simulink model "BFN_02_Thrusters"  (R2019b)
settings: Solver=VariableStepAuto  StartTime=0.0  StopTime=20  MaxStep=0.1  RelTol=1e-3
values from neighbouring files (symbols this model uses):
  MIB = 1e-3    (= 0.001)    [BFN_00_main.m]
  PWM_period = 0.1    [BFN_00_main.m]
  Thr_dir = [0 0 0 0 0 0 0 0 0 0 0 0;     0 0 1 -1 1 -1 0 0 1 -1 1 -1;     1 -1 0 0 0 0 1 -1 0 0 0 0]    [BFN_00_main.m]
  Thr_dist = [17 17 17 17 0 0 -17 -17 -17 -17 0 0;     0 0 0 0 0 0 0 0 0 0 0 0;     0 0 0 0 10 10 0 0 0 0 -10 -10]*1e-2    [BFN_00_main.m]
  Tmax = 500e-6    (= 0.0005)    [BFN_00_main.m]
  Tmin = 10e-6    (= 1e-05)    [BFN_00_main.m]
libraries: simulink x2
settings Model: Creator=Nicola  LastModifiedBy=Nicola

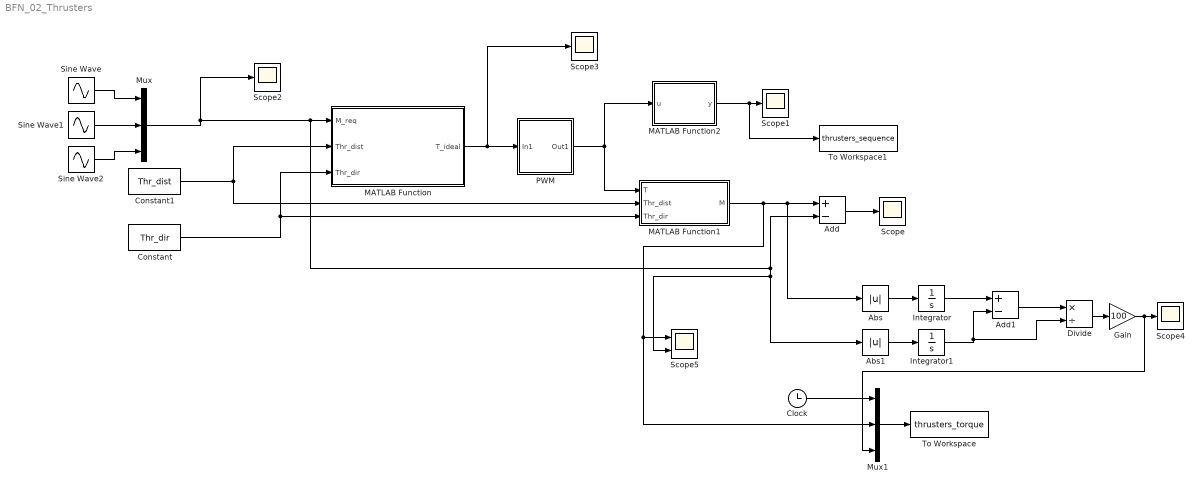
== system BFN_02_Thrusters ==
  Abs : Abs  ZeroCross=off
  Abs1 : Abs  ZeroCross=off
  Add : Sum  Inputs=+-
  Add1 : Sum  Inputs=+-
  Clock : Clock
  Constant : Constant  Value=Thr_dir
  Constant1 : Constant  Value=Thr_dist
  Divide : Product  Inputs=*/
  Gain : Gain  Gain=100
  Integrator : Integrator
  Integrator1 : Integrator
  MATLAB Function : MATLAB Function  TreatAsAtomicUnit=on
  MATLAB Function1 : MATLAB Function  TreatAsAtomicUnit=on
  MATLAB Function2 : MATLAB Function  TreatAsAtomicUnit=on
  Mux : Mux  Inputs=3
  Mux1 : Mux  Inputs=3
  PWM : Subsystem
  Scope{,1..4} (5 alike) : Scope
  Scope5 : Scope  NumInputPorts=2
  Sine Wave : Sin  Amplitude=2*Tmax*0.1*1.2  Frequency=0.3  Phase=60  SampleTime=0
  Sine Wave1 : Sin  Amplitude=2*Tmin*2*0.17  Frequency=0.3  Phase=120+60  SampleTime=0
  Sine Wave2 : Sin  Amplitude=2*Tmin*1.1*0.17  Frequency=0.3  Phase=240+60  SampleTime=0
  To Workspace : ToWorkspace  VariableName=thrusters_torque  SampleTime=-1
      settings: Save2DSignal=2-D array (concatenate along first dimension)
  To Workspace1 : ToWorkspace  VariableName=thrusters_sequence  SampleTime=-1
      settings: Save2DSignal=2-D array (concatenate along first dimension)
  wires:
  Sine Wave1/1 -> Mux/2
  Sine Wave/1 -> Mux/1
  Sine Wave2/1 -> Mux/3
  Constant1/1 -> MATLAB Function1/2(Thr_dist), MATLAB Function/2(Thr_dist)
  Constant/1 -> MATLAB Function/3(Thr_dir), MATLAB Function1/3(Thr_dir)
  MATLAB Function/1(T_ideal) -> PWM/1(In1), Scope3/1
  MATLAB Function2/1(y) -> To Workspace1/1, Scope1/1
  PWM/1(Out1) -> MATLAB Function1/1(T), MATLAB Function2/1(u)
  Mux/1 -> Scope2/1, Abs1/1, Scope5/2, Add/2, MATLAB Function/1(M_req)
  MATLAB Function1/1(M) -> Abs/1, Add/1, Mux1/2, Scope5/1
  Add/1 -> Scope/1
  Abs/1 -> Integrator/1
  Abs1/1 -> Integrator1/1
  Gain/1 -> Mux1/3, Scope4/1
  Integrator/1 -> Add1/1
  Integrator1/1 -> Divide/2, Add1/2
  Add1/1 -> Divide/1
  Divide/1 -> Gain/1
  Mux1/1 -> To Workspace/1
  Clock/1 -> Mux1/1

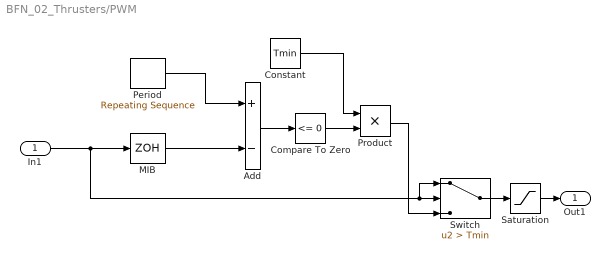
== system BFN_02_Thrusters/PWM ==
  In1 : Inport
  Add : Sum  Inputs=+-
  Compare To Zero : simulink/Logic and Bit Operations/Compare To Zero  relop=<=  OutDataTypeStr=boolean
  Constant : Constant  Value=Tmin
  MIB : ZeroOrderHold  SampleTime=MIB*1.015
  Period : simulink/Sources/Repeating Sequence  rep_seq_t=[0 PWM_period]  rep_seq_y=[0 Tmin]
  Product : Product
  Saturation : Saturate  UpperLimit=Tmax  LowerLimit=-Tmax
  Switch : Switch  Criteria=u2 > Threshold  Threshold=Tmin
  Out1 : Outport
  wires:
  In1/1 -> Switch/1, Switch/2, MIB/1
  Compare To Zero/1 -> Product/2
  Constant/1 -> Product/1
  Add/1 -> Compare To Zero/1
  Period/1 -> Add/1
  MIB/1 -> Add/2
  Switch/1 -> Saturation/1
  Product/1 -> Switch/3
  Saturation/1 -> Out1/1

== matlab function BFN_02_Thrusters/MATLAB Function1 ==
  data: T input; M output; Thr_dist input; Thr_dir input
function M = fcn(T,Thr_dist,Thr_dir)
M1 = cross(Thr_dist,bsxfun(@times,T,Thr_dir));
M = sum(M1,2);

== matlab function BFN_02_Thrusters/MATLAB Function ==
  data: M_req input; T_ideal output; Thr_dist input; Thr_dir input
function T_ideal = fcn(M_req,Thr_dist,Thr_dir)
M0 = cross(Thr_dist,Thr_dir);
M1 = bsxfun(@times, M_req/2,ones(3,12)).*(M0~=0);
T = -1*bsxfun(@rdivide,cross(Thr_dist,M1),dot(Thr_dist,Thr_dist)).*Thr_dir;
T = T.*(T>0);
T_ideal = sum(T,1);

== matlab function BFN_02_Thrusters/MATLAB Function2 ==
  data: u input; y output
function y = fcn(u)

y = u(1:6)';
